simulink model "commented_stateflow"  (R2025b)
settings: Solver=FixedStepDiscrete  StartTime=0.0  StopTime=30  FixedStep=0.1  RelTol=1e-3  EnableMultiTasking=on
settings Model: Creator=ZJO9FE  LastModifiedBy=ZJO9FE
settings SolverCC: AlgebraicLoopSolver=TrustRegion  AutoInsertRateTranBlk=on
settings OptimizationCC: LifeSpan=inf
settings DebuggingCC: UnconnectedInputMsg=warning  UnconnectedOutputMsg=warning  UnconnectedLineMsg=warning  SFUnexpectedBacktrackingDiag=warning  SFNoUnconditionalDefaultTransitionDiag=warning  SFExecutionAtInitializationDiag=none  ArithmeticOperatorsInVariantConditions=warning
settings ModelReferenceCC: EnableRefExpFcnMdlSchedulingChecks=on
settings SFSimCC: SimUseLocalCustomCode=off  CustomCodeUndefinedFunction=UseInterfaceOnly
settings RTWCC: RTWUseLocalCustomCode=off  GPUComputeCapability=3.5  DLArmComputeVersion=19.05
settings CodeAppCC: StateflowObjectComments=on
settings GRTTargetCC: TargetLangStandard=C89/C90 (ANSI)
settings ConfigComp: CovMetricSettings=dw  CovSaveCumulativeToWorkspaceVar=on  CovSaveSingleToWorkspaceVar=on  CovExternalEMLEnable=off

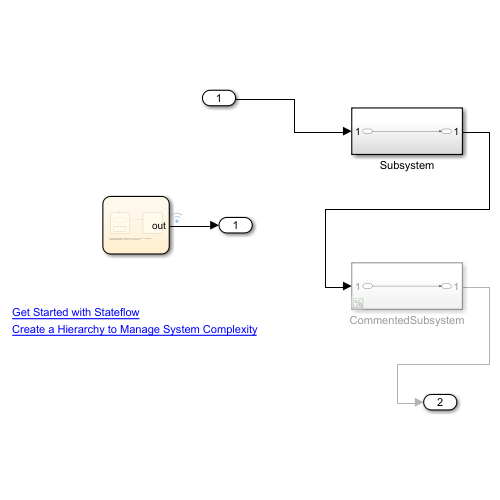
[thumbnail: Simulink's stored preview of the top-level diagram]
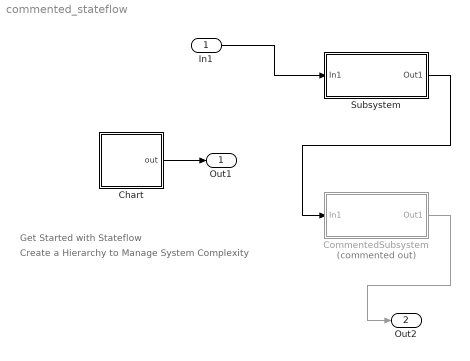
== system commented_stateflow ==
  note: Create a Hierarchy to Manage System Complexity
  note: Get Started with Stateflow
  In1 : Inport
  Chart : Stateflow chart  TreatAsAtomicUnit=on
  CommentedSubsystem : Subsystem  Commented=on
  Subsystem : Subsystem
  Out1 : Outport
  Out2 : Outport  Port=2
  wires:
  Chart/1(out) -> Out1/1
  Subsystem/1(Out1) -> CommentedSubsystem/1(In1)
  CommentedSubsystem/1(Out1) -> Out2/1
  In1/1 -> Subsystem/1(In1)

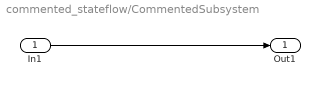
== system commented_stateflow/CommentedSubsystem ==
  In1 : Inport
  Out1 : Outport
  wires:
  In1/1 -> Out1/1

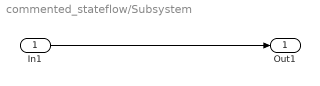
== system commented_stateflow/Subsystem ==
  In1 : Inport
  Out1 : Outport
  wires:
  In1/1 -> Out1/1

== stateflow chart commented_stateflow/Chart ==
  state Run % Parent State
    state High % Child State [commented out]
      entry: out = 10;
    state Low
      entry: out = 1;
    (default) -> High % Child State [commented out]
    Low -> High % Child State [commented out] : after(1,sec)
    High % Child State -> Low [commented out] : after(1,sec)
  state Cooldown
    entry: out = -1;
  note: The Run state contains the child states High and Low . When Run is active, the chart switches between High and Low once per second.
  (default) -> Run % Parent State
  Run % Parent State -> Cooldown : after(10,sec)
  Cooldown -> Run % Parent State [commented out] : after(5,sec)
  data: out output
